simulink model "lab11_test"  (R2024a)
settings: Solver=VariableStepAuto  StartTime=0.0  StopTime=10.0  RelTol=1e-3
values from neighbouring files (symbols this model uses):
  m = 5    [lab3_1.m]    (also in lab43_2.m = 200)
  n = 7    [lab3_1.m]    (also in test.m = length(polynomial1_bin); test_OCMC.m = length(seq1))
settings Model: Creator=QQshnik  LastModifiedBy=QQshnik

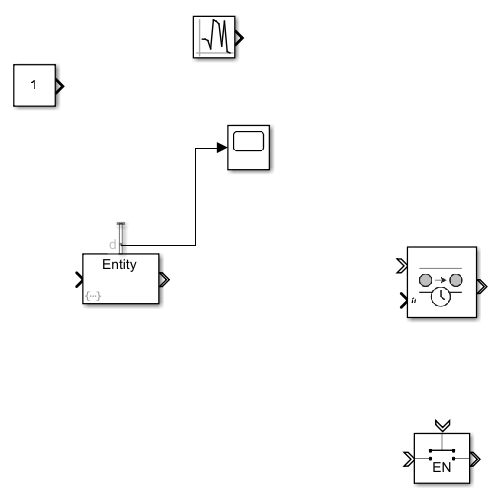
[thumbnail: Simulink's stored preview of the top-level diagram]
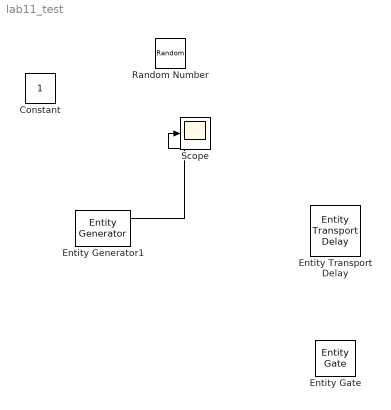
== system lab11_test ==
  Constant : Constant
  Entity Transport Delay : EntityTransportDelay  InputPortMessageModes=m,n  OutputPortMessageModes=m
  Entity Gate : EntityGate  InputPortMessageModes=m,m  OutputPortMessageModes=m
  Entity Generator1 : EntityGenerator  OutputPortMessageModes=n,m  TimeSource=Signal port  GenerateAction=|  AttributeName=nQueries|ArrivalRate|TaskWeight  AttributeInitialValue=20|0.9|2  NumberEntitiesDeparted=on  EntityType=Structured  EntityTypeName=Entity
      | % Параметры
      | nQueries = 20;       % Количество запросов
      | ArrivalRate = 0.9;    % Ставка прибытия (время между запросами)
      | TaskWeight = 2;       % Вес задачи (например, для задания времени обработки)
      | 
      | % Инициализация
      | persistent queryCount;  % Переменная для отслеживания количества запросов
      | if isempty(queryCount)
      |     queryCount = 0;  % Начальное значение счетчика запросов
      | end
      | 
      | % Проверка, нужно ли создавать новый запрос
      | if queryCount < nQueries
      |     queryCount = queryCount + 1;  % Увеличиваем счетчик запросов
      | 
      |     % Генерация новой сущности
      |     entity = createEntity();  % Создание сущности (этот метод создает объект сущности)
      | 
      |     % Присваиваем вес задачи
      |     entity.TaskWeight = TaskWeight;
      | 
      |     % Запланировать следующее прибытие с задержкой по времени
      |     tNextArrival = -log(rand) / ArrivalRate;
      | 
      |     % Возврат сущности с задержкой на основе вычисленного времени
      |     schedule(tNextArrival, entity);
      | end
      settings: InputPortMap=u1  OutputPortMap=o0,o3
  Random Number : RandomNumber  SampleTime=0.1
  Scope : Scope
  wires:
  Entity Generator1/1 -> Scope/1
